simulink model "Env_cpl_buck_online"  (R2023b)
settings: Solver=VariableStepAuto  StartTime=0.0  StopTime=0.4  RelTol=1e-3
PostLoadFcn:
  | , if any(exist('dsrtsu_mdlpostloadfcn', 'file') == [2, 3, 6]), try dsrtsu_mdlpostloadfcn('Execute', bdroot); catch fprintf('Error in PostLoadFcn (dsrtsu_mdlpostloadfcn) for model "%s":\n %s\n', bdroot, lasterr); end, end,
values from neighbouring files (symbols this model uses):
  C = 0.001    [init.m]
  E = 200    [init.m]
  ESO = 0    [init.m]
  fsw = 2e4    (= 20000)    [init.m]
  initial_power = 200    [init.m]
  Kic = 200    [init.m]
  Kiv = 394    [init.m]
  Kpc = 0.02    [init.m]
  Kpv = 3.3    [init.m]
  L = 0.001    [init.m]
  PI = 1    [init.m]
  Switched_power = 800    [init.m]
  Vref = 100    [init.m]
  w0 = 6000    [init.m]
undefined symbols (not defined in the file or in its folder): h, R, W0
libraries: spsSeriesRLCBranchLib x3, spsControlledCurrentSourceLib x1, spsControlledVoltageSourceLib x1, spsCurrentMeasurementLib x1, spsDiodeLib x1, spsMosfetLib x1, spsPWMGeneratorDCDCLib x1, spsVoltageMeasurementLib x1, sps_lib x1
(part 1 of 5)
Description:
  | Standard RTI1006 template.
  | Supported MATLAB version:  R2019a.
settings Model: Tag=RTI1006  DSRTSU_INTERNAL_RTI_VER=540  DSRTSU_INTERNAL_RTI_TYPE=rti1006  RTICANMMDATA=struct('GeneralSetupData',struct('modelroot','E:\WORK\MigrationScripts','generalsettings',struct('filesettings',struct('destfolder',struct('Name','RTICANMM_FILES','Check',1),'buildfolder',struct('Name','.','Check',1),'AbsDestfolder',struct('Name','E:\WORK\MigrationScripts\RTICANMM_FILES'),'AbsBuildfolder',struct('Name','E:\WORK\MigrationScripts'))),'options',struct('addpaths',1,'rmpaths',1,'addtrcexclusion',logical(1),'cannavigator',struct('checkmonitoring',0),'show_usrtrc',0,'use_usrtrc',0),'advanced',struct('options',ones(1,100)),'MPSetup',{{}},'RTI',struct('Type','RTI1006','Ver','7.12','Date','02-May-2019'),'modelname','','block','untitled'))  DSRTSU_INTERNAL_RTIFPGA=130  Creator=user  LastModifiedBy=Dean
settings SolverCC: AlgebraicLoopSolver=TrustRegion
settings DataIOCC: ReturnWorkspaceOutputs=off
settings OptimizationCC: BlockReduction=off  OptimizeBlockIOStorage=off  BufferReuse=off  GlobalBufferReuse=off  ExpressionFolding=off  LocalBlockOutputs=off  OptimizeDataStoreBuffers=off  BusAssignmentInplaceUpdate=off
settings DebuggingCC: UnconnectedInputMsg=warning  UnconnectedOutputMsg=warning  UnconnectedLineMsg=warning  PregeneratedLibrarySubsystemCodeDiagnostic=none  ArithmeticOperatorsInVariantConditions=warning
settings HardwareCC: ProdBitPerPointer=32  ProdBitPerSizeT=32  ProdBitPerPtrDiffT=32  ProdLargestAtomicInteger=Integer  ProdWordSize=32  ProdHWDeviceType=Custom Processor->Custom  TargetIntDivRoundTo=Zero  TargetEndianess=LittleEndian  TargetHWDeviceType=Custom Processor->Custom
settings ModelReferenceCC: EnableRefExpFcnMdlSchedulingChecks=on
settings SFSimCC: SimUseLocalCustomCode=off  MATLABDynamicMemAlloc=off  CustomCodeUndefinedFunction=UseInterfaceOnly
settings RTWCC: Description=dSPACE DS1006 Hardware Platform  SystemTargetFile=rti1006.tlc  MakeCommand=make_rti  TemplateMakefile=rti1006.tmf  RTWUseLocalCustomCode=off  DLArmComputeVersion=19.05
settings CodeAppCC: StateflowObjectComments=on
settings STFCustomTargetCC: TargetLangStandard=C89/C90 (ANSI)  ParMdlRefBuildCompliant=on  MatFileLogging=on  SystemTargetFile=rti1006.tlc
settings GRTTargetCC: TargetLangStandard=C89/C90 (ANSI)  CompOptLevelCompliant=off  ConcurrentExecutionCompliant=off  CombineOutputUpdateFcns=off  CPPClassGenCompliant=off  UseToolchainInfoCompliant=off
settings ConfigComp: CovMetricSettings=dswe

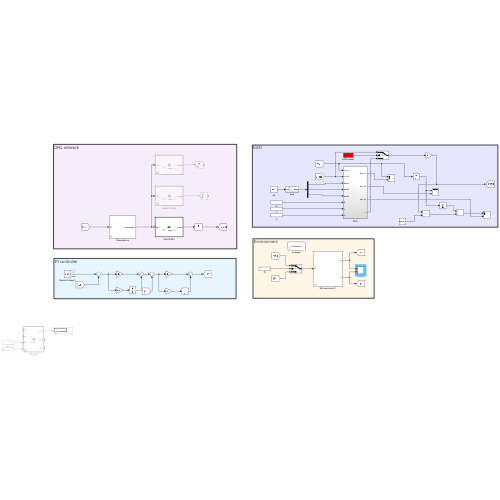
[thumbnail: Simulink's stored preview of the top-level diagram]
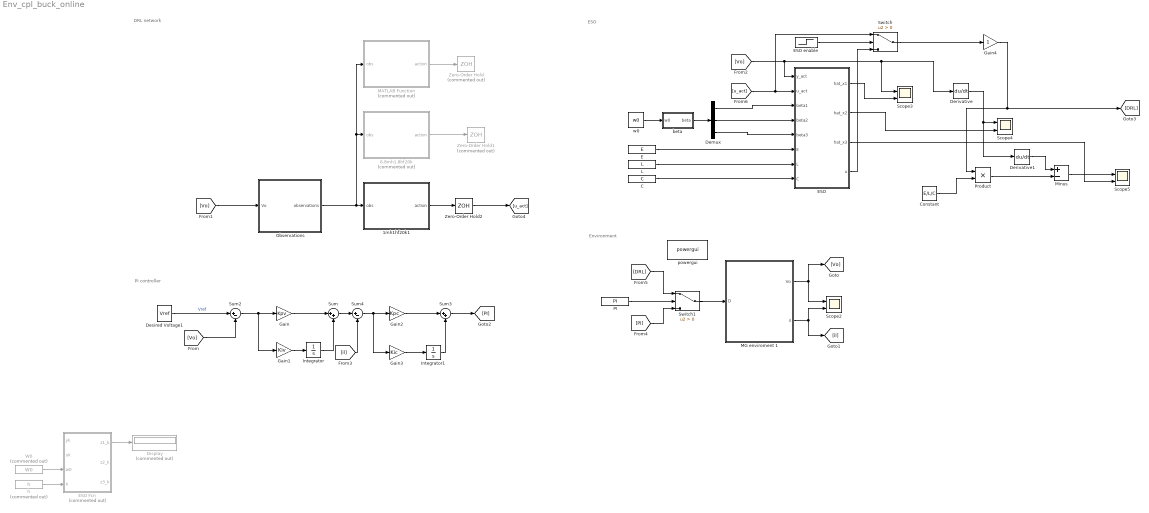
== system Env_cpl_buck_online ==
  note: Environment
  note: DRL network
  note: PI controller
  note: ESO
  1mh1hf20k1 : MATLAB Function  TreatAsAtomicUnit=on
  6.8mh1.8hf20k : MATLAB Function  Commented=on  TreatAsAtomicUnit=on
  C : Constant  Value=C
  Constant : Constant  Value=E/L/C
  Demux : Demux  Outputs=3
  Derivative : Derivative
  Derivative1 : Derivative
  Desired Voltage1 : Constant  Value=Vref
  Display : Display  Commented=on
  E : Constant  Value=E
  ESO : Subsystem
  ESO Fcn : MATLAB Function  Commented=on  TreatAsAtomicUnit=on
  ESO enable : Step  Time=0.01  Before=1  After=ESO  SampleTime=0
  Gain : Gain  Gain=Kpv
  Gain1 : Gain  Gain=Kiv
  Gain2 : Gain  Gain=Kpc
  Gain3 : Gain  Gain=Kic
  Gain4 : Gain
  Integrator : Integrator
  Integrator1 : Integrator
  L : Constant  Value=L
  MATLAB Function : MATLAB Function  Commented=on  TreatAsAtomicUnit=on
  MG enviroment 1 : Subsystem  mask{E=E, L=L, C=C, t1=0.14, t2=0.2, p1=initial_power, p2=Switched_power, fsw=fsw}
      mask prompts: E "Input voltage E (V)"; L "L (H)"; C "C (F)"; t1 "Step time 1"; t2 "Step time2"; p1 "Initial power (W)"; p2 "Switched power (W)"; fsw "Switching frequency (Hz)"
      mask DialogControl ParameterGroupVar Prompt: 参数
  Minus : Sum  Inputs=+-
  Observations : Subsystem  mask{Vref=100}
      mask DialogControl DescTextVar Prompt: Voltage reference
      mask DialogControl ParameterGroupVar Prompt: 参数
  PI : Constant  Value=PI
  Product : Product
  Scope{2..5} (4 alike) : Scope  NumInputPorts=2
  Sum : Sum  Inputs=|++
  Sum2 : Sum  Inputs=|+-
  Sum3 : Sum  Inputs=|++
  Sum4 : Sum  Inputs=|+-
  Switch : Switch  Criteria=u2 > Threshold  SaturateOnIntegerOverflow=off  InputSameDT=off
  Switch1 : Switch  Criteria=u2 > Threshold  SaturateOnIntegerOverflow=off  InputSameDT=off
  W0 : Constant  Commented=on  Value=W0
  Zero-Order Hold : ZeroOrderHold  Commented=on  SampleTime=1/20000
  Zero-Order Hold1 : ZeroOrderHold  Commented=on  SampleTime=1/20000
  Zero-Order Hold2 : ZeroOrderHold  SampleTime=1/20000
  beta : Subsystem
  h : Constant  Commented=on  Value=h
  powergui : sps_lib/powergui  Priority=1  SimulationMode=Continuous  SampleTime=50e-6  frequency=60  Iterations=50  frequencyindice=0  Pbase=100e6  ErrMax=1e-4  UnitsV=kV  UnitsW=MW  buscounter=0  FunctionMessages=off  echomessages=off  EnableUseOfTLC=off  CurrentSourceSwitches=off  DisableSnubberDevices=off  DisableRonSwitches=off  DisableVfSwitches=off  DisplayEquations=off  AutomaticDiscreteSolvers=off  SolverType=Tustin/Backward Euler (TBE)  Interpol=off  ExternalGateDelay=off  methode=off  Ts=100  x0status=blocks  SPID=on  SwTol=0  HookPort=off  NonlinearTolerance=1e-4  nMaxIteration=100  ContinueOnMaxIteration=off  RestoreLinks=warning  ResistiveCurrentMeasurement=off  Frange=[0:2:500]  Ylog=off  Xlog=on  ShowGrid=off  save=off  variable=ZData  structure=0  ZoomFFT=off  StartTime=0.0  cycles=1  DisplayStyle=1  fundamental=60  FreqAxis=off  MaxFrequency=1000  frequencyindicesteady=1  RmsSteady=1  display=off
  w0 : Constant  Value=w0
  wires:
  Observations/1(observations) -> MATLAB Function/1(obs), 6.8mh1.8hf20k/1(obs), 1mh1hf20k1/1(obs)
  MATLAB Function/1(action) -> Zero-Order Hold/1
  6.8mh1.8hf20k/1(action) -> Zero-Order Hold1/1
  1mh1hf20k1/1(action) -> Zero-Order Hold2/1
  E/1 -> ESO/6(E)
  [u_act] -> Switch/1, ESO/2(u_act)
  beta/1(beta) -> Demux/1
  Demux/1 -> ESO/3(beta1)
  Demux/2 -> ESO/4(beta2)
  Demux/3 -> ESO/5(beta3)
  w0/1 -> beta/1(w0)
  L/1 -> ESO/7(L)
  C/1 -> ESO/8(C)
  Gain1/1 -> Integrator/1
  Gain/1 -> Sum/1
  Integrator/1 -> Sum/2
  Desired Voltage1/1 -> Sum2/1  "Vref"
  Sum2/1 -> Gain1/1, Gain/1
  Integrator1/1 -> Sum3/2
  Gain2/1 -> Sum3/1
  Gain3/1 -> Integrator1/1
  Sum/1 -> Sum4/1
  Sum4/1 -> Gain2/1, Gain3/1
  h/1 -> ESO Fcn/4(h)
  W0/1 -> ESO Fcn/3(w0)
  ESO Fcn/1(z1_k) -> Display/1
  ESO enable/1 -> Switch/2
  Sum3/1 -> [PI]
  Switch1/1 -> MG enviroment 1/1(D)
  PI/1 -> Switch1/2
  ESO/1("hat_x1 ") -> Scope3/2
  ESO/2("hat_x2 ") -> Scope4/2
  Derivative/1 -> Derivative1/1, Scope4/1
  Constant/1 -> Product/2
  Product/1 -> Minus/2
  Derivative1/1 -> Minus/1
  ESO/3("hat_x3 ") -> Scope5/2
  Minus/1 -> Scope5/1
  Gain4/1 -> Product/1, [DRL]
  Switch/1 -> Gain4/1
  ESO/4(u) -> Switch/3
  MG enviroment 1/1(Vo) -> Scope2/1, [Vo]
  [Vo] -> Sum2/2
  [Vo] -> Observations/1(Vo)
  [Vo] -> ESO/1(y_act), Derivative/1, Scope3/1
  MG enviroment 1/2(il) -> [il], Scope2/2
  [il] -> Sum4/2
  [PI] -> Switch1/3
  [DRL] -> Switch1/1
  Zero-Order Hold2/1 -> [u_act]

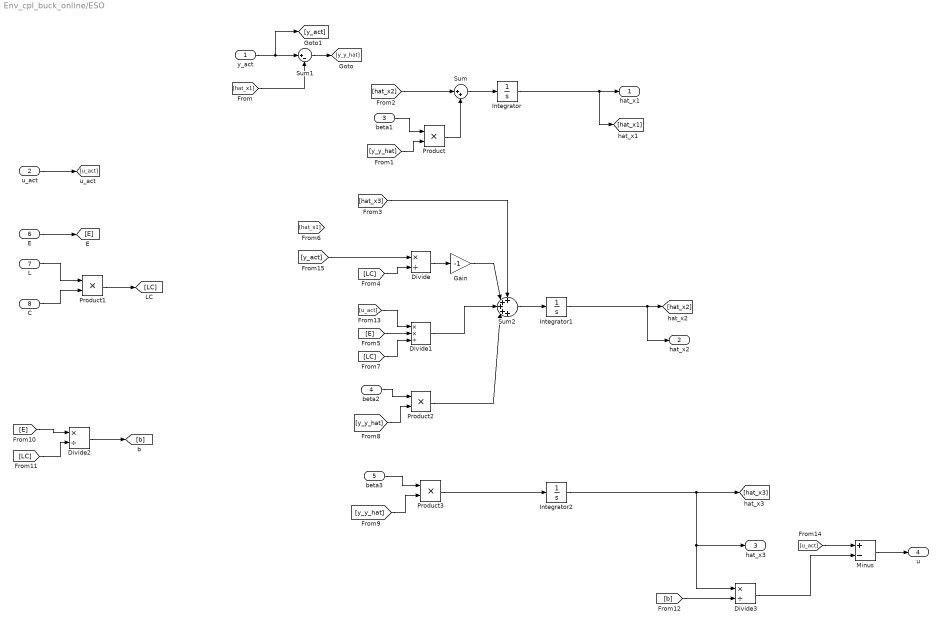
== system Env_cpl_buck_online/ESO ==
  y_act : Inport
  u_act : Inport  Port=2
  beta1 : Inport  Port=3
  beta2 : Inport  Port=4
  beta3 : Inport  Port=5
  E : Inport  Port=6
  L : Inport  Port=7
  C : Inport  Port=8
  Divide : Product  Inputs=*/
  Divide1 : Product  Inputs=**/
  Divide2 : Product  Inputs=*/
  Divide3 : Product  Inputs=*/
  Gain : Gain  Gain=-1
  Integrator : Integrator
  Integrator1 : Integrator
  Integrator2 : Integrator
  Minus : Sum  Inputs=+-
  Product{,1..3} (4 alike) : Product
  Sum : Sum  Inputs=|++
  Sum1 : Sum  Inputs=|+-
  Sum2 : Sum  Inputs=+++++
  "hat_x1 " : Outport  VectorParamsAs1DForOutWhenUnconnected=off
  "hat_x2 " : Outport  Port=2  VectorParamsAs1DForOutWhenUnconnected=off
  "hat_x3 " : Outport  Port=3  VectorParamsAs1DForOutWhenUnconnected=off
  u : Outport  Port=4  VectorParamsAs1DForOutWhenUnconnected=off
  wires:
  y_act/1 -> [y_act], Sum1/1
  [hat_x1] -> Sum1/2
  Sum1/1 -> [y_y_hat]
  beta1/1 -> Product/1
  [y_y_hat] -> Product/2
  Product/1 -> Sum/2
  Sum/1 -> Integrator/1
  [hat_x2] -> Sum/1
  E/1 -> [E]
  L/1 -> Product1/1
  C/1 -> Product1/2
  Product1/1 -> [LC]
  [LC] -> Divide/2
  [E] -> Divide1/2
  [LC] -> Divide1/3
  beta2/1 -> Product2/1
  [y_y_hat] -> Product2/2
  Divide/1 -> Gain/1
  [hat_x3] -> Sum2/1
  Divide1/1 -> Sum2/3
  Product2/1 -> Sum2/4
  Sum2/1 -> Integrator1/1
  beta3/1 -> Product3/1
  [y_y_hat] -> Product3/2
  [E] -> Divide2/1
  [LC] -> Divide2/2
  Divide2/1 -> [b]
  [b] -> Divide3/2
  Integrator/1 -> "hat_x1 "/1, [hat_x1]
  Integrator1/1 -> [hat_x2], "hat_x2 "/1
  Integrator2/1 -> [hat_x3], Divide3/1, "hat_x3 "/1
  Product3/1 -> Integrator2/1
  u_act/1 -> [u_act]
  [u_act] -> Divide1/1
  [u_act] -> Minus/1
  Divide3/1 -> Minus/2
  Minus/1 -> u/1
  Gain/1 -> Sum2/2
  [y_act] -> Divide/1

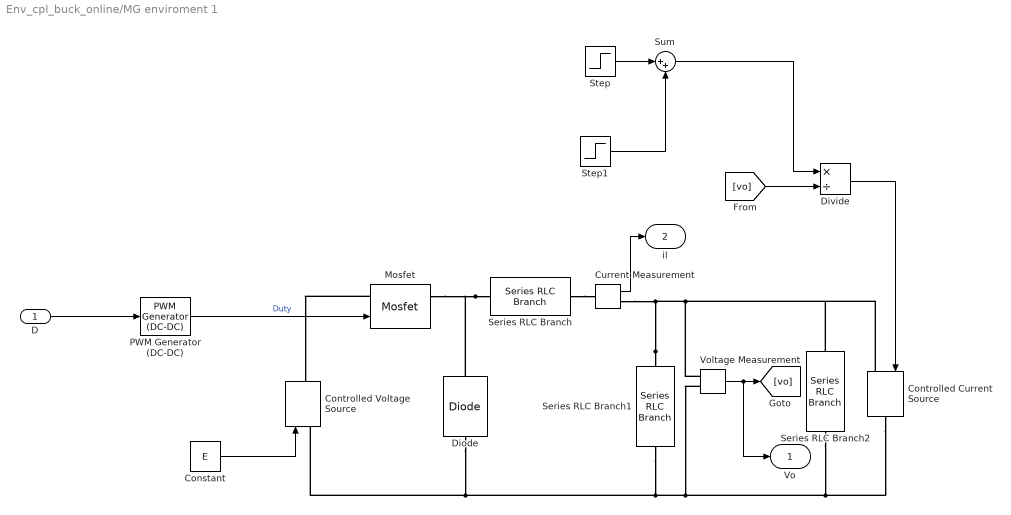
== system Env_cpl_buck_online/MG enviroment 1 ==
  D : Inport
  Constant : Constant  Value=E
  Controlled Current Source : spsControlledCurrentSourceLib/Controlled Current Source  Initialize=on  Source_Type=AC  Amplitude=0  Phase=0  Frequency=0  Measurements=None
  Controlled Voltage Source : spsControlledVoltageSourceLib/Controlled Voltage Source  Initialize=on  Source_Type=AC  Amplitude=0  Phase=0  Frequency=0  Measurements=None
  Current Measurement : spsCurrentMeasurementLib/Current Measurement  PhasorSimulation=off  OutputType=Complex  PSBequivalent=0
  Diode : spsDiodeLib/Diode  Ron=0.001  Lon=0  Vf=0.8  IC=0  UseSnubber=0  Rs=500  Cs=250e-9  Measurements=off
  Divide : Product  Inputs=*/
  Mosfet : spsMosfetLib/Mosfet  Ron=0.1  Lon=0  Rd=0.01  Vfd=0  IC=0  Rs=1e5  Cs=inf  Measurements=on
  PWM Generator (DC-DC) : spsPWMGeneratorDCDCLib/PWM Generator (DC-DC)  Fsw=fsw  Ts=0
  Series RLC Branch : spsSeriesRLCBranchLib/Series RLC Branch  LConnTagsString=__new0  RConnTagsString=__new0  BranchType=L  Resistance=1  Inductance=L  SetiL0=off  InitialCurrent=0  Capacitance=1e-6  Setx0=off  InitialVoltage=0  Measurements=None
  Series RLC Branch1 : spsSeriesRLCBranchLib/Series RLC Branch  LConnTagsString=__new0  RConnTagsString=__new0  BranchType=C  Resistance=1  Inductance=0.002  SetiL0=off  InitialCurrent=0  Capacitance=C  Setx0=on  InitialVoltage=100  Measurements=None
  Series RLC Branch2 : spsSeriesRLCBranchLib/Series RLC Branch  LConnTagsString=__new0  RConnTagsString=__new0  BranchType=R  Resistance=150000  Inductance=R  SetiL0=off  InitialCurrent=0  Capacitance=1e-6  Setx0=off  InitialVoltage=0  Measurements=None
  Step : Step  Time=t1  Before=p1  After=p2  SampleTime=0
  Step1 : Step  Time=t2  After=p1-p2  SampleTime=0
  Sum : Sum  Inputs=|++
  Voltage Measurement : spsVoltageMeasurementLib/Voltage Measurement  PhasorSimulation=off  OutputType=Complex  PSBequivalent=0
  Vo : Outport  VectorParamsAs1DForOutWhenUnconnected=off
  il : Outport  Port=2  VectorParamsAs1DForOutWhenUnconnected=off
  wires:
  Current Measurement/1 -> il/1
  Voltage Measurement/1 -> Vo/1, [vo]
  Divide/1 -> Controlled Current Source/1
  Constant/1 -> Controlled Voltage Source/1
  [vo] -> Divide/2
  Step1/1 -> Sum/2
  Step/1 -> Sum/1
  Sum/1 -> Divide/1
  D/1 -> PWM Generator (DC-DC)/1
  PWM Generator (DC-DC)/1 -> Mosfet/1  "Duty"
  connections:
  Controlled Current Source/RConn1 -- Diode/LConn1 -- Controlled Voltage Source/LConn1 -- Series RLC Branch1/RConn1 -- Voltage Measurement/LConn2 -- Series RLC Branch2/RConn1
  Series RLC Branch1/LConn1 -- Current Measurement/RConn1 -- Series RLC Branch2/LConn1 -- Controlled Current Source/LConn1 -- Voltage Measurement/LConn1
  Series RLC Branch/LConn1 -- Mosfet/RConn1 -- Diode/RConn1
  Series RLC Branch/RConn1 -- Current Measurement/LConn1
  Mosfet/LConn1 -- Controlled Voltage Source/RConn1

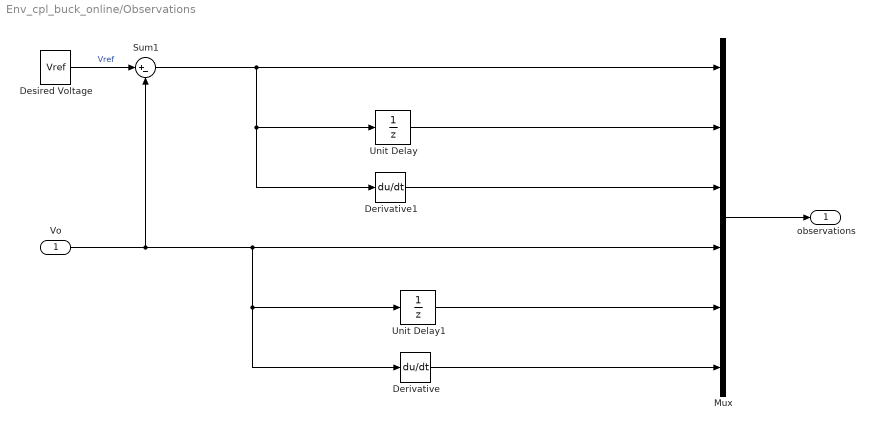
== system Env_cpl_buck_online/Observations ==
  Vo : Inport
  Derivative : Derivative
  Derivative1 : Derivative
  Desired Voltage : Constant  Value=Vref
  Mux : Mux  Inputs=6
  Sum1 : Sum  Inputs=|+-  SaturateOnIntegerOverflow=on
  Unit Delay : UnitDelay  SampleTime=-1  HasFrameUpgradeWarning=on
  Unit Delay1 : UnitDelay  SampleTime=-1  HasFrameUpgradeWarning=on
  observations : Outport  VectorParamsAs1DForOutWhenUnconnected=off
  wires:
  Mux/1 -> observations/1
  Derivative1/1 -> Mux/3
  Unit Delay/1 -> Mux/2
  Derivative/1 -> Mux/6
  Unit Delay1/1 -> Mux/5
  Vo/1 -> Sum1/2, Unit Delay1/1, Derivative/1, Mux/4
  Sum1/1 -> Unit Delay/1, Derivative1/1, Mux/1
  Desired Voltage/1 -> Sum1/1  "Vref"

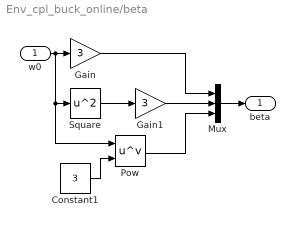
== system Env_cpl_buck_online/beta ==
  w0 : Inport
  Constant1 : Constant  Value=3
  Gain : Gain  Gain=3
  Gain1 : Gain  Gain=3
  Mux : Mux  Inputs=3
  Pow : Math  Operator=pow  RndMeth=Zero
  Square : Math  Operator=square
  beta : Outport
  wires:
  Constant1/1 -> Pow/2
  Square/1 -> Gain1/1
  w0/1 -> Pow/1, Square/1, Gain/1
  Gain/1 -> Mux/1
  Gain1/1 -> Mux/2
  Pow/1 -> Mux/3
  Mux/1 -> beta/1
